simulink model "assgn_1"  (R2021a)
settings: Solver=VariableStepAuto  StartTime=0.0  StopTime=10.0  RelTol=1e-3
values from neighbouring files (symbols this model uses):
  c1 = 100    [assgn_1_const.m.m]
  c2 = 1000    [assgn_1_const.m.m]
  k1 = 1e4    (= 10000)    [assgn_1_const.m.m]
  k2 = 1e5    (= 100000)    [assgn_1_const.m.m]
  m1 = 10    [assgn_1_const.m.m]
  m2 = 100    [assgn_1_const.m.m]
settings Model: Creator=Aastik  LastModifiedBy=Aastik

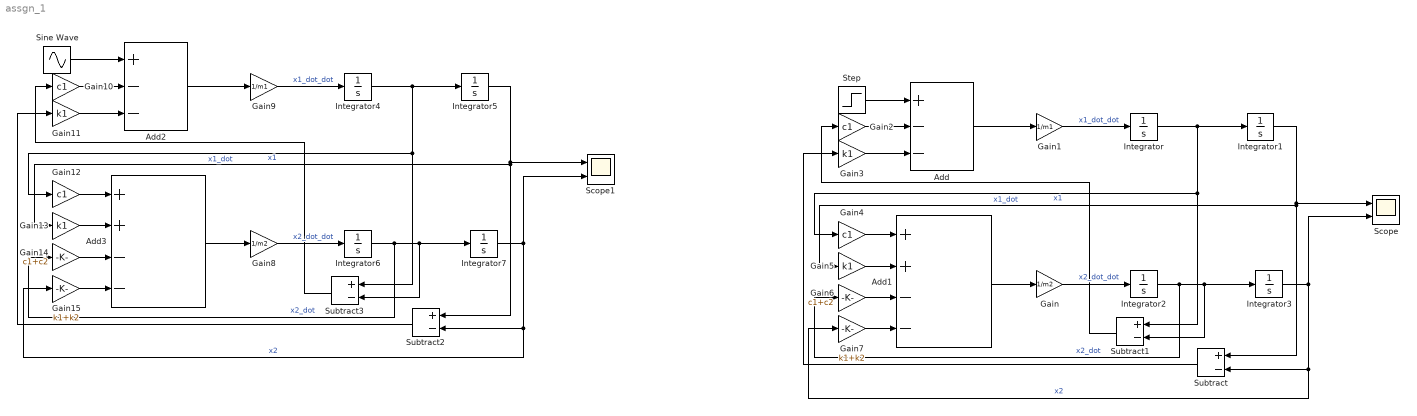
== system assgn_1 ==
  Add : Sum  Inputs=+--
  Add1 : Sum  Inputs=++--
  Add2 : Sum  Inputs=+--
  Add3 : Sum  Inputs=++--
  Gain : Gain  Gain=1/m2
  Gain1 : Gain  Gain=1/m1
  Gain{2,4,10,12} (4 alike) : Gain  Gain=c1
  Gain{3,5,11,13} (4 alike) : Gain  Gain=k1
  Gain14 : Gain  Gain=c1+c2
  Gain15 : Gain  Gain=k1+k2
  Gain6 : Gain  Gain=c1+c2
  Gain7 : Gain  Gain=k1+k2
  Gain8 : Gain  Gain=1/m2
  Gain9 : Gain  Gain=1/m1
  Integrator{,1..7} (8 alike) : Integrator
  Scope : Scope  NumInputPorts=2
  Scope1 : Scope  NumInputPorts=2
  Sine Wave : Sin  Amplitude=3  Frequency=10  SampleTime=0
  Step : Step  Time=5  SampleTime=0
  Subtract{,1..3} (4 alike) : Sum  Inputs=+-
  wires:
  Gain1/1 -> Integrator/1  "x1_dot_dot"
  Integrator/1 -> Gain4/1, Subtract1/1, Integrator1/1  "x1_dot"
  Integrator1/1 -> Subtract/1, Gain5/1, Scope/1  "x1"
  Gain/1 -> Integrator2/1  "x2_dot_dot"
  Integrator2/1 -> Gain6/1, Subtract1/2, Integrator3/1  "x2_dot"
  Integrator3/1 -> Scope/2, Gain7/1, Subtract/2  "x2"
  Gain2/1 -> Add/2
  Gain3/1 -> Add/3
  Subtract/1 -> Gain3/1
  Subtract1/1 -> Gain2/1
  Add/1 -> Gain1/1
  Gain4/1 -> Add1/1
  Add1/1 -> Gain/1
  Gain5/1 -> Add1/2
  Gain6/1 -> Add1/3
  Gain7/1 -> Add1/4
  Step/1 -> Add/1
  Sine Wave/1 -> Add2/1
  Gain13/1 -> Add3/2
  Gain14/1 -> Add3/3
  Gain15/1 -> Add3/4
  Add2/1 -> Gain9/1
  Gain12/1 -> Add3/1
  Gain11/1 -> Add2/3
  Subtract3/1 -> Gain10/1
  Gain8/1 -> Integrator6/1  "x2_dot_dot"
  Gain9/1 -> Integrator4/1  "x1_dot_dot"
  Gain10/1 -> Add2/2
  Integrator7/1 -> Scope1/2, Gain15/1, Subtract2/2  "x2"
  Integrator4/1 -> Gain12/1, Subtract3/1, Integrator5/1  "x1_dot"
  Subtract2/1 -> Gain11/1
  Integrator6/1 -> Gain14/1, Subtract3/2, Integrator7/1  "x2_dot"
  Add3/1 -> Gain8/1
  Integrator5/1 -> Subtract2/1, Gain13/1, Scope1/1  "x1"
